simulink model "UnicycleModel"  (R2016b)
settings: Solver=ode45  StartTime=0.0  StopTime=11  FixedStep=0.1  MaxStep=1  RelTol=1e-3
settings Model: Creator=danielefontanelli  LastModifiedBy=giacomo2
settings SolverCC: ZeroCrossAlgorithm=Adaptive

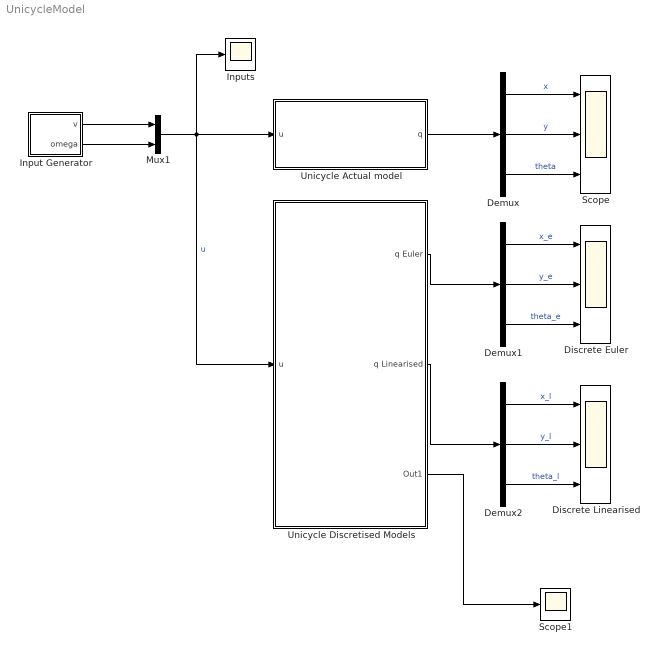
== system UnicycleModel ==
  Demux : Demux  Outputs=3
  Demux1 : Demux  Outputs=3
  Demux2 : Demux  Outputs=3
  Discrete Euler : Scope  NumInputPorts=3
  Discrete Linearised : Scope  NumInputPorts=3
  Input Generator : Subsystem
  Inputs : Scope
  Mux1 : Mux  Inputs=2
  Scope : Scope  NumInputPorts=3
  Scope1 : Scope
  Unicycle Actual model : Subsystem
  Unicycle Discretised Models : Subsystem
  wires:
  Mux1/1 -> Unicycle Discretised Models/1(u), Unicycle Actual model/1(u), Inputs/1  "u"
  Demux/2 -> Scope/2  "y"
  Demux/1 -> Scope/1  "x"
  Demux/3 -> Scope/3  "theta"
  Input Generator/1(v) -> Mux1/1
  Input Generator/2(omega) -> Mux1/2
  Unicycle Actual model/1(q) -> Demux/1
  Unicycle Discretised Models/1(q Euler) -> Demux1/1
  Demux1/1 -> Discrete Euler/1  "x_e"
  Demux1/2 -> Discrete Euler/2  "y_e"
  Demux1/3 -> Discrete Euler/3  "theta_e"
  Unicycle Discretised Models/2(q Linearised) -> Demux2/1
  Demux2/1 -> Discrete Linearised/1  "x_l"
  Demux2/2 -> Discrete Linearised/2  "y_l"
  Demux2/3 -> Discrete Linearised/3  "theta_l"
  Unicycle Discretised Models/3(Out1) -> Scope1/1

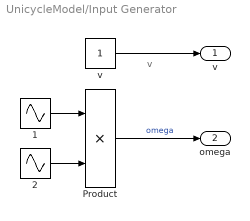
== system UnicycleModel/Input Generator ==
  note: v
  1 : Sin  Amplitude=2  Frequency=2*pi/10  SampleTime=0
  2 : Sin  Frequency=2*pi/2  SampleTime=0
  Product : Product
  "v " : Constant
  v : Outport
  omega : Outport  Port=2
  wires:
  2/1 -> Product/2
  1/1 -> Product/1
  "v "/1 -> v/1
  Product/1 -> omega/1  "omega"

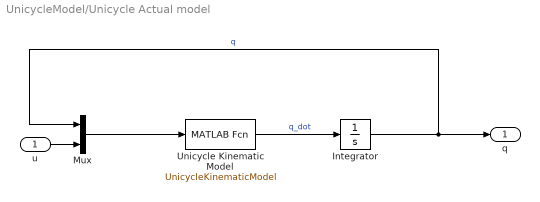
== system UnicycleModel/Unicycle Actual model ==
  u : Inport
  Integrator : Integrator  InitialCondition="[0  0  0]"
  Mux : Mux  Inputs=2
  Unicycle Kinematic Model : MATLABFcn  MATLABFcn=UnicycleKinematicModel
  q : Outport
  wires:
  u/1 -> Mux/2
  Integrator/1 -> q/1, Mux/1  "q"
  Unicycle Kinematic Model/1 -> Integrator/1  "q_dot"
  Mux/1 -> Unicycle Kinematic Model/1

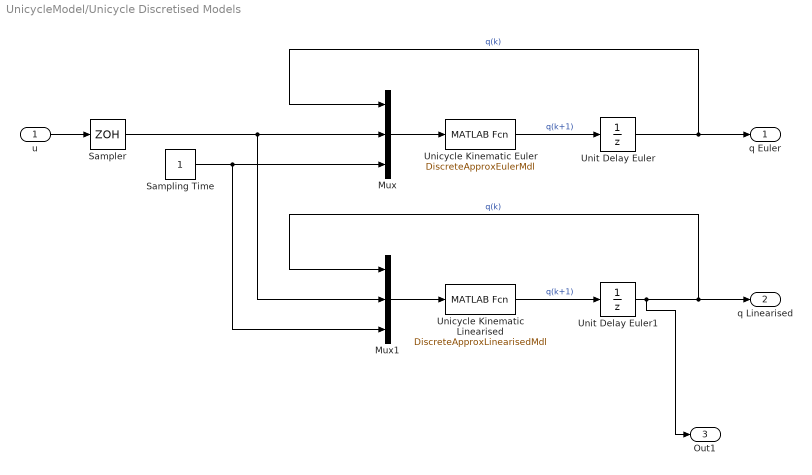
== system UnicycleModel/Unicycle Discretised Models ==
  u : Inport
  Mux : Mux  Inputs=3
  Mux1 : Mux  Inputs=3
  Sampler : ZeroOrderHold
  Sampling Time : Constant
  Unicycle Kinematic Euler : MATLABFcn  MATLABFcn=DiscreteApproxEulerMdl  SampleTime=1
  Unicycle Kinematic Linearised : MATLABFcn  MATLABFcn=DiscreteApproxLinearisedMdl  SampleTime=1
  Unit Delay Euler : UnitDelay  InitialCondition="[0  0  0]"  SampleTime=-1
  Unit Delay Euler1 : UnitDelay  InitialCondition="[0  0  0]"  SampleTime=-1
  q Euler : Outport
  q Linearised : Outport  Port=2
  Out1 : Outport  Port=3
  wires:
  u/1 -> Sampler/1
  Unit Delay Euler/1 -> q Euler/1, Mux/1  "q(k)"
  Unicycle Kinematic Euler/1 -> Unit Delay Euler/1  "q(k+1)"
  Mux/1 -> Unicycle Kinematic Euler/1
  Unit Delay Euler1/1 -> Out1/1, q Linearised/1, Mux1/1  "q(k)"
  Unicycle Kinematic Linearised/1 -> Unit Delay Euler1/1  "q(k+1)"
  Mux1/1 -> Unicycle Kinematic Linearised/1
  Sampling Time/1 -> Mux1/3, Mux/3
  Sampler/1 -> Mux1/2, Mux/2
